simulink model "CollingSystemSIMULINK"  (R2024b)
settings: Solver=VariableStepAuto  StartTime=0.0  StopTime=20.0  RelTol=1e-3
libraries: fuzblock x1

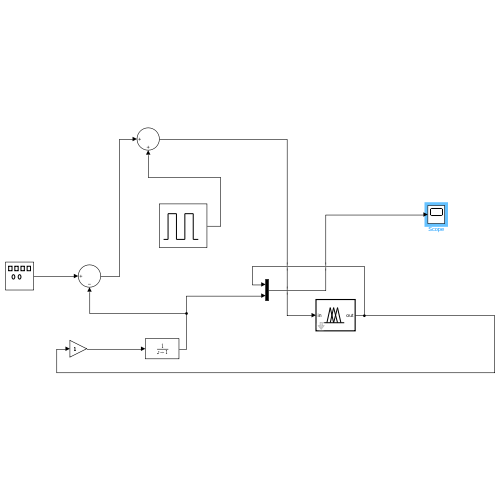
[thumbnail: Simulink's stored preview of the top-level diagram]
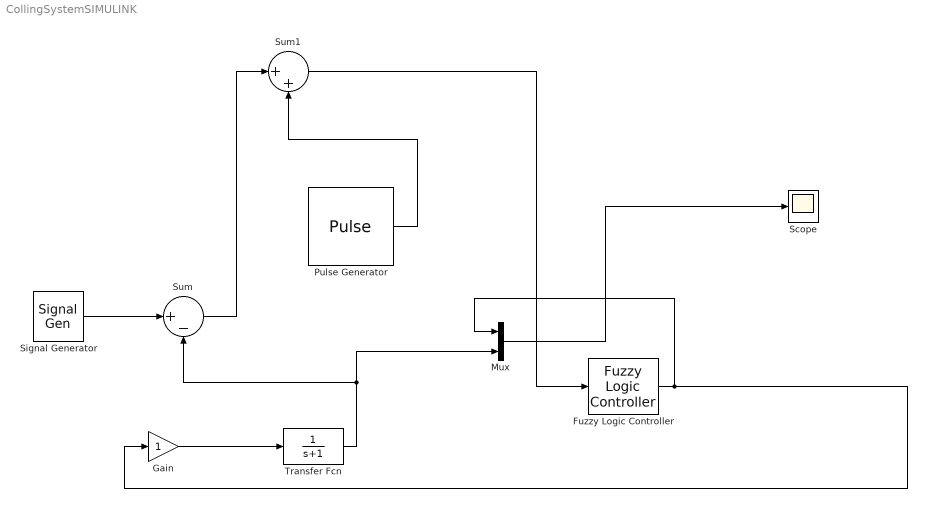
== system CollingSystemSIMULINK ==
  Fuzzy Logic Controller : fuzblock/Fuzzy Logic  Controller  FIS='CoolingFuzzyController.fis'  OutputSampleNumber=101  DataType=double  FuzzifiedInputs=off  RuleFiringStrengths=off  RuleOutputs=off  AggregatedOutputs=off  SimulateUsing=Interpreted execution  OutOfRangeInputValueMessage=warning  NoRuleFiredMessage=warning  EmptyOutputFuzzySetMessage=warning
  Gain : Gain
  Mux : Mux  Inputs=2
  Pulse Generator : DiscretePulseGenerator  PulseType=Time based  Amplitude=3  Period=10  PulseWidth=50
  Scope : Scope
  Signal Generator : SignalGenerator  Amplitude=0  Units=rad/sec
  Sum : Sum  Inputs=|+-
  Sum1 : Sum  Inputs=|++
  Transfer Fcn : TransferFcn  Denominator=[1 1]
  wires:
  Signal Generator/1 -> Sum/1
  Fuzzy Logic Controller/1 -> Mux/1, Gain/1
  Gain/1 -> Transfer Fcn/1
  Transfer Fcn/1 -> Sum/2, Mux/2
  Sum/1 -> Sum1/1
  Pulse Generator/1 -> Sum1/2
  Sum1/1 -> Fuzzy Logic Controller/1
  Mux/1 -> Scope/1
